simulink model "modelo_SIRV"  (R2019b)
settings: Solver=VariableStepAuto  StartTime=0.0  StopTime=100  RelTol=1e-3
undefined symbols (not defined in the file): beta, gamma, I0, nu, R0, S0
settings Model: Creator=lucia  LastModifiedBy=lucia

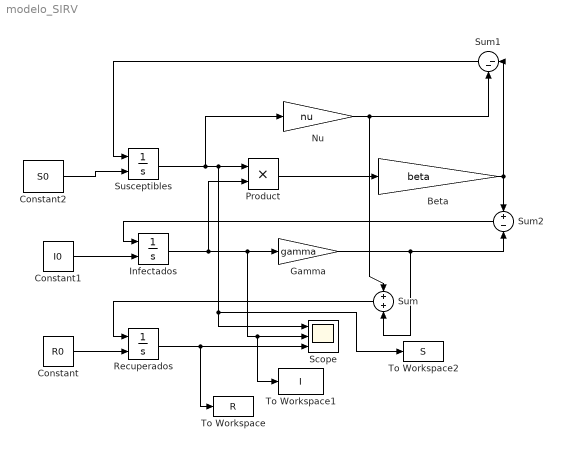
== system modelo_SIRV ==
  Beta : Gain  Gain=beta
  Constant : Constant  Value=R0
  Constant1 : Constant  Value=I0
  Constant2 : Constant  Value=S0
  Gamma : Gain  Gain=gamma
  Infectados : Integrator  InitialConditionSource=external
  Nu : Gain  Gain=nu
  Product : Product
  Recuperados : Integrator  InitialConditionSource=external
  Scope : Scope  NumInputPorts=3
  Sum : Sum
  Sum1 : Sum  Inputs=|--
  Sum2 : Sum  Inputs=+-
  Susceptibles : Integrator  InitialConditionSource=external
  To Workspace : ToWorkspace  VariableName=R  SaveFormat=Structure With Time  SampleTime=-1
  To Workspace1 : ToWorkspace  VariableName=I  SaveFormat=Structure With Time  SampleTime=-1
  To Workspace2 : ToWorkspace  VariableName=S  SaveFormat=Structure With Time  SampleTime=-1
  wires:
  Infectados/1 -> Product/2, To Workspace1/1, Scope/2, Gamma/1
  Product/1 -> Beta/1
  Susceptibles/1 -> To Workspace2/1, Scope/1, Product/1, Nu/1
  Constant1/1 -> Infectados/2
  Constant2/1 -> Susceptibles/2
  Beta/1 -> Sum1/1, Sum2/1
  Nu/1 -> Sum1/2, Sum/1
  Sum1/1 -> Susceptibles/1
  Gamma/1 -> Sum/2, Sum2/2
  Sum2/1 -> Infectados/1
  Constant/1 -> Recuperados/2
  Sum/1 -> Recuperados/1
  Recuperados/1 -> To Workspace/1, Scope/3
